simulink model "20240109_HVDCMMCInterconnection"  (R2023b)
settings: Solver=FixedStepDiscrete  StartTime=0.0  StopTime=2  FixedStep=Ts_Power  RelTol=1e-4  EnableMultiTasking=on
PreLoadFcn:
  | HVDCMMCInterconnectionParam
StartFcn:
  | tic
StopFcn:
  | toc
values from neighbouring files (symbols this model uses):
  C_PM = 1.758e-3    (= 0.001758)    [HVDCMMCInterconnectionParam.m]
  Cg = 50e-9    (= 5e-08)    [HVDCMMCInterconnectionParam.m]
  D_R = 0.001    [HVDCMMCInterconnectionParam.m]
  D_Rs = 1e8    (= 100000000)    [HVDCMMCInterconnectionParam.m]
  D_Vf = 0    [HVDCMMCInterconnectionParam.m]
  Fnom = 50    [HVDCMMCInterconnectionParam.m]
  HRM = 2    [HVDCMMCInterconnectionParam.m]
  Ki_Ireg = 6    [HVDCMMCInterconnectionParam.m]
  Ki_Preg = 1.0    (= 1)    [HVDCMMCInterconnectionParam.m]
  Ki_Qreg = 1.0    (= 1)    [HVDCMMCInterconnectionParam.m]
  Ki_VDCreg = 100    [HVDCMMCInterconnectionParam.m]
  Kp_Ireg = 0.6    [HVDCMMCInterconnectionParam.m]
  Kp_Preg = 0.5/3    (= 0.166666666667)    [HVDCMMCInterconnectionParam.m]
  Kp_Qreg = 0.5/3    (= 0.166666666667)    [HVDCMMCInterconnectionParam.m]
  Kp_VDCreg = 4    [HVDCMMCInterconnectionParam.m]
  L_cable = 15e-3    (= 0.015)    [HVDCMMCInterconnectionParam.m]
  Larm = Larm_pu*(Zb_ac/(2*pi*Fnom))    [HVDCMMCInterconnectionParam.m]
  Lff = Larm_pu/2    (= 0.075)    [HVDCMMCInterconnectionParam.m]
  Limits_Ireg = [ 2.0  -2.0]    [HVDCMMCInterconnectionParam.m]
  Limits_Preg = [ 1.2, 0.8 ]    [HVDCMMCInterconnectionParam.m]
  Limits_Qreg = [ 0.25, -0.25 ]    [HVDCMMCInterconnectionParam.m]
  Limits_VDCreg = [ 2.0  -2.0]    [HVDCMMCInterconnectionParam.m]
  Lxfo = 0.12    [HVDCMMCInterconnectionParam.m]
  Nb_PM = 36    [HVDCMMCInterconnectionParam.m]
  Pnom = 1000e6    (= 1000000000)    [HVDCMMCInterconnectionParam.m]
  R_cable = 0.5    [HVDCMMCInterconnectionParam.m]
  R_startup = 400    [HVDCMMCInterconnectionParam.m]
  Rarm = Rarm_pu*Zb_ac    [HVDCMMCInterconnectionParam.m]
  Rff = Rarm_pu/2    (= 0.00075)    [HVDCMMCInterconnectionParam.m]
  Rg = 100    [HVDCMMCInterconnectionParam.m]
  Rxfo = 0.003    [HVDCMMCInterconnectionParam.m]
  Slope_Pref = 0.5    [HVDCMMCInterconnectionParam.m]
  Slope_Qref = 0.5    [HVDCMMCInterconnectionParam.m]
  Slope_Vdc_ref = Vnom_dc/5    (= 128000)    [HVDCMMCInterconnectionParam.m]
  Tbrk1_On = 0.1    [HVDCMMCInterconnectionParam.m]
  Tbrk2_On = 1.0    (= 1)    [HVDCMMCInterconnectionParam.m]
  Tdeblock = 1.5    [HVDCMMCInterconnectionParam.m]
  Tfault = 9999    [HVDCMMCInterconnectionParam.m]
  Ton_Converter2 = 4    [HVDCMMCInterconnectionParam.m]
  Ton_PQreg = 4    [HVDCMMCInterconnectionParam.m]
  Ton_VDCreg = 1.5    [HVDCMMCInterconnectionParam.m]
  Ts = Ts_Control    (= 4e-05)    [HVDCMMCInterconnectionParam.m]
  Ts_Control = 40e-6    (= 4e-05)    [HVDCMMCInterconnectionParam.m]
  Ts_Power = 20e-6    (= 2e-05)    [HVDCMMCInterconnectionParam.m]
  Vb_ac = sqrt(2/3)*Vnom_sec    [HVDCMMCInterconnectionParam.m]
  Vb_dc = Vnom_dc    (= 640000)    [HVDCMMCInterconnectionParam.m]
  Vc0_PM = 0    [HVDCMMCInterconnectionParam.m]
  Vnom_dc = 640e3    (= 640000)    [HVDCMMCInterconnectionParam.m]
  Vnom_prim = 400e3    (= 400000)    [HVDCMMCInterconnectionParam.m]
  Vnom_sec = 333e3    (= 333000)    [HVDCMMCInterconnectionParam.m]
  w = 2*pi*Fnom    (= 314.159265359)    [HVDCMMCInterconnectionParam.m]
undefined symbols (not defined in the file or in its folder): DiscIntNeverNeededParam, gcbh, Pcc, S, sps_AC, sps_ACDC2, sps_rtmsupport
libraries: simulink x48, spsControlledVoltageSourceLib x30, spsCurrentMeasurementLib x30, MMC_Lib x30, spsDiodeLib x20, spsSeriesRLCBranchLib x14, powerlib_extras x12, spsVoltageMeasurementLib x12, spsSecondOrderFilterLib x8, spsabctodq0Lib x8, spsGroundLib x7, spsMeanLib x4
(part 6 of 9)

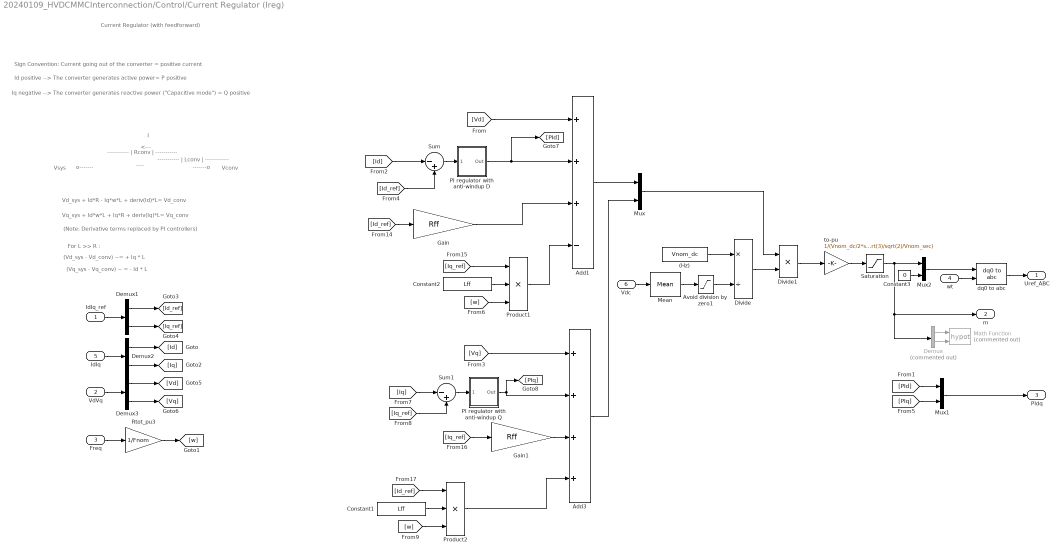
== system 20240109_HVDCMMCInterconnection/Control/Current Regulator (Ireg) ==
  note: -----------
      | | Lconv |
      | ------------
  note: <---
  note: -------o
  note: Vconv
  note: ----
  note: -----------
      | | Rconv |
      | -----------
  note: For L >> R :
  note: (Vq_sys - Vq_conv) ~ = - Id * L
  note: (Vd_sys - Vd_conv) ~= + Iq * L
  note: Id positive --> The converter generates active power= P positive
  note: Iq negative --> The converter generates reactive power ("Capacitive mode") = Q positive
  note: Sign Convention: Current going out of the converter = positive current
  note: Current Regulator
      | (with feedforward)
  note: Vq_sys + Id*w*L + Iq*R + deriv(Iq)*L= Vq_conv
  note: Vd_sys + Id*R - Iq*w*L + deriv(Id)*L= Vd_conv
  note: (Note: Derivative terms replaced by PI controllers)
  note: Vsys
  note: o-------
  note: I
  IdIq_ref : Inport  PortDimensions=2
  VdVq : Inport  Port=2  PortDimensions=2
  Freq : Inport  Port=3  PortDimensions=1
  wt : Inport  Port=4  PortDimensions=1
  IdIq : Inport  Port=5  PortDimensions=2
  Vdc : Inport  Port=6  PortDimensions=1
  " (Hz)" : Constant  Value=Vnom_dc  SampleTime=Ts
  Add1 : Sum  Inputs=+++-
  Add3 : Sum  Inputs=++++
  Avoid division by zero1 : Saturate  UpperLimit=Vnom_dc*1.25  LowerLimit=Vnom_dc*0.75
  Constant1 : Constant  Value=Lff  SampleTime=Ts_Control
  Constant2 : Constant  Value=Lff  SampleTime=Ts_Control
  Constant3 : Constant  Value=0  SampleTime=Ts
  Demux : Demux  Commented=on  Outputs=2
  Demux1 : Demux  Outputs=2
  Demux2 : Demux  Outputs=2
  Demux3 : Demux  Outputs=2
  Divide : Product  Inputs=*/
  Divide1 : Product  Inputs=**
  Gain : Gain  Gain=Rff
  Gain1 : Gain  Gain=Rff
  Math Function : Math  Commented=on  Operator=hypot  SignedPower=on
  Mean : spsMeanLib/Mean  Freq=Fnom/3  Vinit=Vnom_dc  Ts=Ts
  Mux : Mux  Inputs=2
  Mux1 : Mux  Inputs=2
  Mux2 : Mux  Inputs=[2 1]
  PI regulator with anti-windup D : Subsystem  DialogController=POWERSYS.PowerSysDialog  mask(Discrete PI Controller){Kp=Kp_Ireg, Ki=Ki_Ireg, Par_Limits=Limits_Ireg, Init=0, Ts=Ts}
      mask prompts: Kp "Proportional gain (Kp):"; Ki "Integral gain (Ki):"; Par_Limits "Output limits: [ Upper   Lower ]"; Init "Output initial value:"; Ts "Sample time:"
      mask help: This block implements a discrete PI controller.
      mask init:
      | UpperLimit=Par_Limits(1);
      | LowerLimit=Par_Limits(2);
      | power_initmask();
      mask Help: This block is part of a subset of blocks in the Extras library that does not have documentation associated with it, other than the block mask description.
      mask Display: disp('PI');
  PI regulator with anti-windup Q : Subsystem  DialogController=POWERSYS.PowerSysDialog  mask(Discrete PI Controller){Kp=Kp_Ireg, Ki=Ki_Ireg, Par_Limits=Limits_Ireg, Init=0, Ts=Ts}
      mask prompts: Kp "Proportional gain (Kp):"; Ki "Integral gain (Ki):"; Par_Limits "Output limits: [ Upper   Lower ]"; Init "Output initial value:"; Ts "Sample time:"
      mask help: This block implements a discrete PI controller.
      mask init:
      | UpperLimit=Par_Limits(1);
      | LowerLimit=Par_Limits(2);
      | power_initmask();
      mask Help: This block is part of a subset of blocks in the Extras library that does not have documentation associated with it, other than the block mask description.
      mask Display: disp('PI');
  Product1 : Product  Inputs=3  RndMeth=Zero
  Product2 : Product  Inputs=3  RndMeth=Zero
  Rtot_pu3 : Gain  Gain=1/Fnom  SaturateOnIntegerOverflow=on  OutDataTypeStr=Inherit: Same as input  ParamDataTypeStr=Inherit: Same as input
  Saturation : Saturate  UpperLimit=Limits_Ireg(1)  LowerLimit=Limits_Ireg(2)
  Sum : Sum  Inputs=|-+
  Sum1 : Sum  Inputs=|-+
  dq0 to abc : spsdq0toabcLib/dq0 to abc  Alignment=90 degrees behind phase A axis
  to-pu : Gain  Gain=1/(Vnom_dc/2*sqrt(3)/sqrt(2)/Vnom_sec)
  Uref_ABC : Outport
  m : Outport  Port=2
  PIdq : Outport  Port=3
  wires:
  wt/1 -> dq0 to abc/2
  to-pu/1 -> Saturation/1
  Mux/1 -> Divide1/1
  dq0 to abc/1 -> Uref_ABC/1
  Divide/1 -> Divide1/2
  Mean/1 -> Avoid division by zero1/1
  Divide1/1 -> to-pu/1
  " (Hz)"/1 -> Divide/1
  Vdc/1 -> Mean/1
  Avoid division by zero1/1 -> Divide/2
  Mux1/1 -> PIdq/1
  Constant3/1 -> Mux2/2
  Mux2/1 -> dq0 to abc/1
  Demux/2 -> Math Function/2
  Demux/1 -> Math Function/1
  Saturation/1 -> Mux2/1, m/1, Demux/1
  PI regulator with anti-windup D/1(Out) -> [PId], Add1/2
  PI regulator with anti-windup Q/1(Out) -> [PIq], Add3/2
  [Vd] -> Add1/1
  Product1/1 -> Add1/4
  Gain/1 -> Add1/3
  Gain1/1 -> Add3/3
  Product2/1 -> Add3/4
  [Vq] -> Add3/1
  Demux2/1 -> [Id]
  IdIq/1 -> Demux2/1
  [Id_ref] -> Product2/1
  [Iq_ref] -> Gain1/1
  [Iq_ref] -> Product1/1
  [Id_ref] -> Gain/1
  [Id] -> Sum/1
  [Iq] -> Sum1/1
  Demux2/2 -> [Iq]
  [PIq] -> Mux1/2
  [PId] -> Mux1/1
  [w] -> Product1/3
  Constant2/1 -> Product1/2
  [w] -> Product2/3
  Constant1/1 -> Product2/2
  [Iq_ref] -> Sum1/2
  Sum1/1 -> PI regulator with anti-windup Q/1(Error)
  [Id_ref] -> Sum/2
  Sum/1 -> PI regulator with anti-windup D/1(Error)
  VdVq/1 -> Demux3/1
  Demux3/2 -> [Vq]
  Demux3/1 -> [Vd]
  IdIq_ref/1 -> Demux1/1
  Demux1/2 -> [Iq_ref]
  Demux1/1 -> [Id_ref]
  Rtot_pu3/1 -> [w]
  Freq/1 -> Rtot_pu3/1
  Add1/1 -> Mux/1
  Add3/1 -> Mux/2

== system 20240109_HVDCMMCInterconnection/Control/DC Voltage Regulator (VDCreg) ==
  note: VDC Regulator
  Vdc_ref : Inport  PortDimensions=1
  On : Inport  Port=2  PortDimensions=1
  Vdc_meas : Inport  Port=3  PortDimensions=1
  Discrete-Time Integrator : DiscreteIntegrator  SampleTime=Ts  LimitOutput=on  UpperSaturationLimit=Limits_VDCreg(1)  LowerSaturationLimit=Limits_VDCreg(2)  ICPrevOutput=DiscIntNeverNeededParam  ICPrevScaledInput=DiscIntNeverNeededParam
  Product : Product  RndMeth=Zero
  Product1 : Product  RndMeth=Zero
  Rtot_pu2 : Gain  Gain=1/Vnom_dc  SaturateOnIntegerOverflow=on  OutDataTypeStr=Inherit: Same as input  ParamDataTypeStr=Inherit: Same as input
  Saturation2 : Saturate  UpperLimit=Limits_VDCreg(1)  LowerLimit=Limits_VDCreg(2)  SampleTime=Ts
  Sum : Sum  Inputs=|+-
  Sum6 : Sum  InputSameDT=on  SaturateOnIntegerOverflow=on  SampleTime=Ts  OutDataTypeStr=Inherit: Same as first input
  Switch1 : Switch  Criteria=u2 ~= 0  Threshold=0.5  OutDataTypeStr=double  SaturateOnIntegerOverflow=off  InputSameDT=off
  VdcNom_SM : Constant  Value=Kp_VDCreg
  VdcNom_SM1 : Constant  Value=Ki_VDCreg
  Zero-Order Hold : ZeroOrderHold  SampleTime=Ts
  Id_ref : Outport
  wires:
  Rtot_pu2/1 -> Product/2, Product1/2
  Saturation2/1 -> Id_ref/1
  VdcNom_SM/1 -> Product1/1
  Product/1 -> Discrete-Time Integrator/1
  Product1/1 -> Zero-Order Hold/1
  VdcNom_SM1/1 -> Product/1
  Sum6/1 -> Saturation2/1
  Discrete-Time Integrator/1 -> Sum6/2
  Zero-Order Hold/1 -> Sum6/1
  Vdc_ref/1 -> Sum/2, Switch1/3
  Switch1/1 -> Sum/1
  On/1 -> Switch1/2
  Sum/1 -> Rtot_pu2/1
  Vdc_meas/1 -> Switch1/1

== system 20240109_HVDCMMCInterconnection/Control/PLL, Measurements and Transformation ==
  note: P (pu) = Vd*Id + Vq*Iq
  note: Q (pu) = Vq*Id - Vd*Iq
  note: P positive = Converter generates active power (Inverter Mode)
  note: Q positive = Converter generates reactive power (Capacitive Mode)
  Vabc : Inport  PortDimensions=3
  Iabc : Inport  Port=2  PortDimensions=3
  Add : Sum  Inputs=1
  Demux : Demux  Outputs=2
  Discrete Mean value : powerlib_extras/Discrete Measurements/Discrete  Mean value  Freq=Fnom  Vinit=0  Ts=Ts
  Discrete Mean value1 : powerlib_extras/Discrete Measurements/Discrete  Mean value  Freq=Fnom  Vinit=0  Ts=Ts
  I->pu2 : Gain  Gain=sqrt(3)*Vnom_sec/sqrt(2)/Pnom  SaturateOnIntegerOverflow=on  OutDataTypeStr=Inherit: Same as input  ParamDataTypeStr=Inherit: Same as input
  PLL (3ph) : spsPLL3phLib/PLL (3ph)  Fmin=0.9*Fnom  Par_Init=[0, Fnom]  ParK=[180, 3200, 1]  TcD=1e-4  MaxRateChangeFreq=12  FilterCutOffFreq=25  Ts=Ts  AGC=on
  Product : Product  RndMeth=Zero
  Product1 : Product  RndMeth=Zero
  Second-Order Filter : spsSecondOrderFilterLib/Second-Order Filter  FilterType=Lowpass  Fo=Fn_filter  Zeta=Zeta_filter  Ts=Ts  Initialize=off  Vac_Init="[0,  0,  60]"  Vdc_Init=0  PlotResponse=off  FreqRange=[0, 500, 1]
  Second-Order Filter1 : spsSecondOrderFilterLib/Second-Order Filter  FilterType=Lowpass  Fo=Fn_filter  Zeta=Zeta_filter  Ts=Ts  Initialize=off  Vac_Init="[0,  0,  60]"  Vdc_Init=0  PlotResponse=off  FreqRange=[0, 500, 1]
  Selector3 : Selector  InputPortWidth=2  IndexOptions=Index vector (dialog)  Indices=[2 1]  OutputSizes=1
  Selector4 : Selector  InputPortWidth=3  IndexOptions=Index vector (dialog)  Indices=[1 2]  OutputSizes=1
  Selector5 : Selector  InputPortWidth=3  IndexOptions=Index vector (dialog)  Indices=[1 2]  OutputSizes=1
  Subtract : Sum  Inputs=+-
  V->pu1 : Gain  Gain=1/(Vnom_sec/sqrt(3)*sqrt(2))  SaturateOnIntegerOverflow=on  OutDataTypeStr=Inherit: Same as input  ParamDataTypeStr=Inherit: Same as input
  abc to dq0 : spsabctodq0Lib/abc to dq0  Alignment=90 degrees behind phase A axis
  abc to dq1 : spsabctodq0Lib/abc to dq0  Alignment=90 degrees behind phase A axis
  Freq : Outport
  wt : Outport  Port=2
  IdIq : Outport  Port=3
  P : Outport  Port=4
  Q : Outport  Port=5
  VdVq : Outport  Port=6
  wires:
  Selector3/1 -> Product1/1
  Discrete Mean value1/1 -> Q/1
  Discrete Mean value/1 -> P/1
  Second-Order Filter/1 -> VdVq/1, Product/1, Selector3/1
  Second-Order Filter1/1 -> IdIq/1, Product1/2, Product/2
  Product/1 -> Add/1
  Product1/1 -> Demux/1
  Demux/1 -> Subtract/1
  Demux/2 -> Subtract/2
  Add/1 -> Discrete Mean value/1
  Subtract/1 -> Discrete Mean value1/1
  abc to dq0/1 -> Selector4/1
  PLL (3ph)/1 -> Freq/1
  V->pu1/1 -> abc to dq0/1, PLL (3ph)/1
  Vabc/1 -> V->pu1/1
  PLL (3ph)/2 -> wt/1, abc to dq1/2, abc to dq0/2
  Iabc/1 -> I->pu2/1
  abc to dq1/1 -> Selector5/1
  I->pu2/1 -> abc to dq1/1
  Selector4/1 -> Second-Order Filter/1
  Selector5/1 -> Second-Order Filter1/1

== system 20240109_HVDCMMCInterconnection/Control/Reactive Power Regulator ==
  note: Reactive Power Regulator
  note: If PLL sync on Vprim --> Vq=0 --> Id = P/Vd et Iq = -1.0 * Q/Vd
  note: Q (pu) = Vq*Id - Vd*Iq (valid only for balanced & harmonics-free values)
  note: P (pu) = Vd*Id + Vq*Iq (Zero-sequence is not taken into account)
  On : Inport  PortDimensions=1
  Qref : Inport  Port=2  PortDimensions=1
  Qmes : Inport  Port=3  PortDimensions=1
  VdVq_mes : Inport  Port=4  PortDimensions=2
  Add2 : Sum
  Discrete Mean value1 : powerlib_extras/Discrete Measurements/Discrete  Mean value  Freq=Fnom  Vinit=0  Ts=Ts
  Discrete-Time Integrator : DiscreteIntegrator  SampleTime=Ts  LimitOutput=on  UpperSaturationLimit=Limits_Qreg(1)  LowerSaturationLimit=Limits_Qreg(2)  ICPrevOutput=DiscIntNeverNeededParam  ICPrevScaledInput=DiscIntNeverNeededParam
  Divide : Product  Inputs=*/
  Product : Product  RndMeth=Zero
  Product1 : Product  RndMeth=Zero
  Rtot_pu1 : Gain  Gain=-1  SaturateOnIntegerOverflow=on  OutDataTypeStr=Inherit: Same as input  ParamDataTypeStr=Inherit: Same as input
  Rtot_pu2 : Gain  Gain=-1  SaturateOnIntegerOverflow=on  OutDataTypeStr=Inherit: Same as input  ParamDataTypeStr=Inherit: Same as input
  Saturation : Saturate  UpperLimit=Limits_Qreg(1)  LowerLimit=Limits_Qreg(2)
  Saturation1 : Saturate  UpperLimit=2  LowerLimit=1e-6
  Saturation2 : Saturate  UpperLimit=Limits_Qreg(1)  LowerLimit=Limits_Qreg(2)
  Selector : Selector  InputPortWidth=2  IndexOptions=Index vector (dialog)  Indices=[1]  OutputSizes=1
  Sum : Sum  Inputs=|-+
  Sum6 : Sum  InputSameDT=on  SaturateOnIntegerOverflow=on  SampleTime=Ts  OutDataTypeStr=Inherit: Same as first input
  Switch1 : Switch  Criteria=u2 ~= 0  Threshold=0.5  OutDataTypeStr=double  SaturateOnIntegerOverflow=off  InputSameDT=off
  VdcNom_SM : Constant  Value=Kp_Qreg
  VdcNom_SM1 : Constant  Value=Ki_Qreg
  Zero-Order Hold : ZeroOrderHold  SampleTime=Ts
  Iq_ref : Outport
  wires:
  Saturation2/1 -> Rtot_pu1/1
  Saturation/1 -> Iq_ref/1
  Rtot_pu2/1 -> Add2/2
  Rtot_pu1/1 -> Add2/1
  Sum6/1 -> Saturation2/1
  Switch1/1 -> Product1/2, Product/2
  Sum/1 -> Switch1/1
  On/1 -> Switch1/2
  Add2/1 -> Saturation/1
  Product/1 -> Discrete-Time Integrator/1
  Product1/1 -> Zero-Order Hold/1
  VdcNom_SM/1 -> Product1/1
  VdcNom_SM1/1 -> Product/1
  Discrete-Time Integrator/1 -> Sum6/2
  Zero-Order Hold/1 -> Sum6/1
  Discrete Mean value1/1 -> Saturation1/1
  Saturation1/1 -> Divide/2
  Divide/1 -> Rtot_pu2/1
  Selector/1 -> Discrete Mean value1/1
  VdVq_mes/1 -> Selector/1
  Qmes/1 -> Sum/1
  Qref/1 -> Divide/1, Switch1/3, Sum/2

== system 20240109_HVDCMMCInterconnection/Control1/Active Power Regulator (Preg) ==
  note: Active Power Regulator
  Pmeas : Inport  PortDimensions=1
  Pref : Inport  Port=2  PortDimensions=1  SampleTime=Ts
  On : Inport  Port=3  PortDimensions=1  SampleTime=Ts
  Discrete-Time Integrator : DiscreteIntegrator  InitialCondition=1  SampleTime=Ts  LimitOutput=on  UpperSaturationLimit=Limits_Preg(1)  LowerSaturationLimit=Limits_Preg(2)  ICPrevOutput=DiscIntNeverNeededParam  ICPrevScaledInput=DiscIntNeverNeededParam
  Product : Product  RndMeth=Zero
  Product1 : Product  RndMeth=Zero
  Product2 : Product
  Saturation2 : Saturate  UpperLimit=Limits_Preg(1)  LowerLimit=Limits_Preg(2)  SampleTime=Ts
  Sum : Sum  Inputs=|+-
  Sum6 : Sum  InputSameDT=on  SaturateOnIntegerOverflow=on  SampleTime=Ts  OutDataTypeStr=Inherit: Same as first input
  Switch1 : Switch  Criteria=u2 ~= 0  Threshold=0.5  OutDataTypeStr=double  SaturateOnIntegerOverflow=off  InputSameDT=off
  VdcNom_SM : Constant  Value=Kp_Preg  SampleTime=Ts
  VdcNom_SM1 : Constant  Value=Ki_Preg  SampleTime=Ts
  VdcNom_SM2 : Constant  Value=Vnom_dc  SampleTime=Ts
  Zero-Order Hold : ZeroOrderHold  SampleTime=Ts
  Vdc_ref : Outport  SampleTime=Ts
  wires:
  Product2/1 -> Vdc_ref/1
  VdcNom_SM2/1 -> Product2/2
  Pmeas/1 -> Switch1/1
  On/1 -> Switch1/2
  Switch1/1 -> Sum/1
  Pref/1 -> Switch1/3, Sum/2
  Zero-Order Hold/1 -> Sum6/1
  Discrete-Time Integrator/1 -> Sum6/2
  Sum6/1 -> Saturation2/1
  VdcNom_SM1/1 -> Product/1
  Product1/1 -> Zero-Order Hold/1
  Product/1 -> Discrete-Time Integrator/1
  VdcNom_SM/1 -> Product1/1
  Saturation2/1 -> Product2/1
  Sum/1 -> Product1/2, Product/2

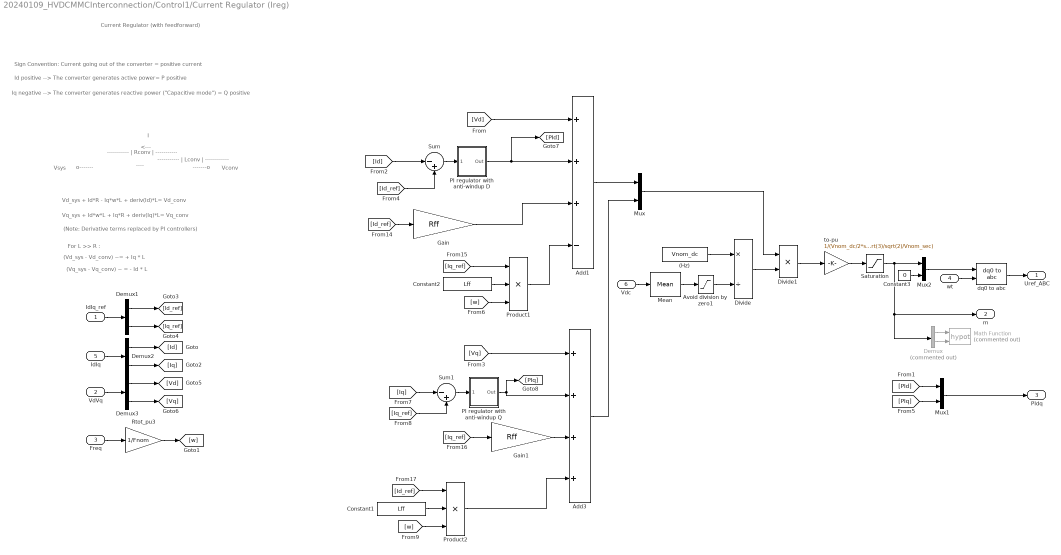
== system 20240109_HVDCMMCInterconnection/Control1/Current Regulator (Ireg) ==
  note: -----------
      | | Lconv |
      | ------------
  note: <---
  note: -------o
  note: Vconv
  note: ----
  note: -----------
      | | Rconv |
      | -----------
  note: For L >> R :
  note: (Vq_sys - Vq_conv) ~ = - Id * L
  note: (Vd_sys - Vd_conv) ~= + Iq * L
  note: Id positive --> The converter generates active power= P positive
  note: Iq negative --> The converter generates reactive power ("Capacitive mode") = Q positive
  note: Sign Convention: Current going out of the converter = positive current
  note: Current Regulator
      | (with feedforward)
  note: Vq_sys + Id*w*L + Iq*R + deriv(Iq)*L= Vq_conv
  note: Vd_sys + Id*R - Iq*w*L + deriv(Id)*L= Vd_conv
  note: (Note: Derivative terms replaced by PI controllers)
  note: Vsys
  note: o-------
  note: I
  IdIq_ref : Inport  PortDimensions=2
  VdVq : Inport  Port=2  PortDimensions=2
  Freq : Inport  Port=3  PortDimensions=1
  wt : Inport  Port=4  PortDimensions=1
  IdIq : Inport  Port=5  PortDimensions=2
  Vdc : Inport  Port=6  PortDimensions=1
  " (Hz)" : Constant  Value=Vnom_dc  SampleTime=Ts
  Add1 : Sum  Inputs=+++-
  Add3 : Sum  Inputs=++++
  Avoid division by zero1 : Saturate  UpperLimit=Vnom_dc*1.25  LowerLimit=Vnom_dc*0.75
  Constant1 : Constant  Value=Lff  SampleTime=Ts_Control
  Constant2 : Constant  Value=Lff  SampleTime=Ts_Control
  Constant3 : Constant  Value=0  SampleTime=Ts
  Demux : Demux  Commented=on  Outputs=2
  Demux1 : Demux  Outputs=2
  Demux2 : Demux  Outputs=2
  Demux3 : Demux  Outputs=2
  Divide : Product  Inputs=*/
  Divide1 : Product  Inputs=**
  Gain : Gain  Gain=Rff
  Gain1 : Gain  Gain=Rff
  Math Function : Math  Commented=on  Operator=hypot  SignedPower=on
  Mean : spsMeanLib/Mean  Freq=Fnom/3  Vinit=Vnom_dc  Ts=Ts
  Mux : Mux  Inputs=2
  Mux1 : Mux  Inputs=2
  Mux2 : Mux  Inputs=[2 1]
  PI regulator with anti-windup D : Subsystem  DialogController=POWERSYS.PowerSysDialog  mask(Discrete PI Controller){Kp=Kp_Ireg, Ki=Ki_Ireg, Par_Limits=Limits_Ireg, Init=0, Ts=Ts}
      mask prompts: Kp "Proportional gain (Kp):"; Ki "Integral gain (Ki):"; Par_Limits "Output limits: [ Upper   Lower ]"; Init "Output initial value:"; Ts "Sample time:"
      mask help: This block implements a discrete PI controller.
      mask init:
      | UpperLimit=Par_Limits(1);
      | LowerLimit=Par_Limits(2);
      | power_initmask();
      mask Help: This block is part of a subset of blocks in the Extras library that does not have documentation associated with it, other than the block mask description.
      mask Display: disp('PI');
  PI regulator with anti-windup Q : Subsystem  DialogController=POWERSYS.PowerSysDialog  mask(Discrete PI Controller){Kp=Kp_Ireg, Ki=Ki_Ireg, Par_Limits=Limits_Ireg, Init=0, Ts=Ts}
      mask prompts: Kp "Proportional gain (Kp):"; Ki "Integral gain (Ki):"; Par_Limits "Output limits: [ Upper   Lower ]"; Init "Output initial value:"; Ts "Sample time:"
      mask help: This block implements a discrete PI controller.
      mask init:
      | UpperLimit=Par_Limits(1);
      | LowerLimit=Par_Limits(2);
      | power_initmask();
      mask Help: This block is part of a subset of blocks in the Extras library that does not have documentation associated with it, other than the block mask description.
      mask Display: disp('PI');
  Product1 : Product  Inputs=3  RndMeth=Zero
  Product2 : Product  Inputs=3  RndMeth=Zero
  Rtot_pu3 : Gain  Gain=1/Fnom  SaturateOnIntegerOverflow=on  OutDataTypeStr=Inherit: Same as input  ParamDataTypeStr=Inherit: Same as input
  Saturation : Saturate  UpperLimit=Limits_Ireg(1)  LowerLimit=Limits_Ireg(2)
  Sum : Sum  Inputs=|-+
  Sum1 : Sum  Inputs=|-+
  dq0 to abc : spsdq0toabcLib/dq0 to abc  Alignment=90 degrees behind phase A axis
  to-pu : Gain  Gain=1/(Vnom_dc/2*sqrt(3)/sqrt(2)/Vnom_sec)
  Uref_ABC : Outport
  m : Outport  Port=2
  PIdq : Outport  Port=3
  wires:
  wt/1 -> dq0 to abc/2
  to-pu/1 -> Saturation/1
  Mux/1 -> Divide1/1
  dq0 to abc/1 -> Uref_ABC/1
  Divide/1 -> Divide1/2
  Mean/1 -> Avoid division by zero1/1
  Divide1/1 -> to-pu/1
  " (Hz)"/1 -> Divide/1
  Vdc/1 -> Mean/1
  Avoid division by zero1/1 -> Divide/2
  Mux1/1 -> PIdq/1
  Constant3/1 -> Mux2/2
  Mux2/1 -> dq0 to abc/1
  Demux/2 -> Math Function/2
  Demux/1 -> Math Function/1
  Saturation/1 -> Mux2/1, m/1, Demux/1
  PI regulator with anti-windup D/1(Out) -> [PId], Add1/2
  PI regulator with anti-windup Q/1(Out) -> [PIq], Add3/2
  [Vd] -> Add1/1
  Product1/1 -> Add1/4
  Gain/1 -> Add1/3
  Gain1/1 -> Add3/3
  Product2/1 -> Add3/4
  [Vq] -> Add3/1
  Demux2/1 -> [Id]
  IdIq/1 -> Demux2/1
  [Id_ref] -> Product2/1
  [Iq_ref] -> Gain1/1
  [Iq_ref] -> Product1/1
  [Id_ref] -> Gain/1
  [Id] -> Sum/1
  [Iq] -> Sum1/1
  Demux2/2 -> [Iq]
  [PIq] -> Mux1/2
  [PId] -> Mux1/1
  [w] -> Product1/3
  Constant2/1 -> Product1/2
  [w] -> Product2/3
  Constant1/1 -> Product2/2
  [Iq_ref] -> Sum1/2
  Sum1/1 -> PI regulator with anti-windup Q/1(Error)
  [Id_ref] -> Sum/2
  Sum/1 -> PI regulator with anti-windup D/1(Error)
  VdVq/1 -> Demux3/1
  Demux3/2 -> [Vq]
  Demux3/1 -> [Vd]
  IdIq_ref/1 -> Demux1/1
  Demux1/2 -> [Iq_ref]
  Demux1/1 -> [Id_ref]
  Rtot_pu3/1 -> [w]
  Freq/1 -> Rtot_pu3/1
  Add1/1 -> Mux/1
  Add3/1 -> Mux/2

== system 20240109_HVDCMMCInterconnection/Control1/DC Voltage Regulator (VDCreg) ==
  note: VDC Regulator
  Vdc_ref : Inport  PortDimensions=1
  On : Inport  Port=2  PortDimensions=1
  Vdc_meas : Inport  Port=3  PortDimensions=1
  Discrete-Time Integrator : DiscreteIntegrator  SampleTime=Ts  LimitOutput=on  UpperSaturationLimit=Limits_VDCreg(1)  LowerSaturationLimit=Limits_VDCreg(2)  ICPrevOutput=DiscIntNeverNeededParam  ICPrevScaledInput=DiscIntNeverNeededParam
  Product : Product  RndMeth=Zero
  Product1 : Product  RndMeth=Zero
  Rtot_pu2 : Gain  Gain=1/Vnom_dc  SaturateOnIntegerOverflow=on  OutDataTypeStr=Inherit: Same as input  ParamDataTypeStr=Inherit: Same as input
  Saturation2 : Saturate  UpperLimit=Limits_VDCreg(1)  LowerLimit=Limits_VDCreg(2)  SampleTime=Ts
  Sum : Sum  Inputs=|+-
  Sum6 : Sum  InputSameDT=on  SaturateOnIntegerOverflow=on  SampleTime=Ts  OutDataTypeStr=Inherit: Same as first input
  Switch1 : Switch  Criteria=u2 ~= 0  Threshold=0.5  OutDataTypeStr=double  SaturateOnIntegerOverflow=off  InputSameDT=off
  VdcNom_SM : Constant  Value=Kp_VDCreg
  VdcNom_SM1 : Constant  Value=Ki_VDCreg
  Zero-Order Hold : ZeroOrderHold  SampleTime=Ts
  Id_ref : Outport
  wires:
  Rtot_pu2/1 -> Product/2, Product1/2
  Saturation2/1 -> Id_ref/1
  VdcNom_SM/1 -> Product1/1
  Product/1 -> Discrete-Time Integrator/1
  Product1/1 -> Zero-Order Hold/1
  VdcNom_SM1/1 -> Product/1
  Sum6/1 -> Saturation2/1
  Discrete-Time Integrator/1 -> Sum6/2
  Zero-Order Hold/1 -> Sum6/1
  Vdc_ref/1 -> Sum/2, Switch1/3
  Switch1/1 -> Sum/1
  On/1 -> Switch1/2
  Sum/1 -> Rtot_pu2/1
  Vdc_meas/1 -> Switch1/1

== system 20240109_HVDCMMCInterconnection/Control1/PLL, Measurements and Transformation ==
  note: P (pu) = Vd*Id + Vq*Iq
  note: Q (pu) = Vq*Id - Vd*Iq
  note: P positive = Converter generates active power (Inverter Mode)
  note: Q positive = Converter generates reactive power (Capacitive Mode)
  Vabc : Inport  PortDimensions=3
  Iabc : Inport  Port=2  PortDimensions=3
  Add : Sum  Inputs=1
  Demux : Demux  Outputs=2
  Discrete Mean value : powerlib_extras/Discrete Measurements/Discrete  Mean value  Freq=Fnom  Vinit=0  Ts=Ts
  Discrete Mean value1 : powerlib_extras/Discrete Measurements/Discrete  Mean value  Freq=Fnom  Vinit=0  Ts=Ts
  I->pu2 : Gain  Gain=sqrt(3)*Vnom_sec/sqrt(2)/Pnom  SaturateOnIntegerOverflow=on  OutDataTypeStr=Inherit: Same as input  ParamDataTypeStr=Inherit: Same as input
  PLL (3ph) : spsPLL3phLib/PLL (3ph)  Fmin=0.9*Fnom  Par_Init=[0, Fnom]  ParK=[180, 3200, 1]  TcD=1e-4  MaxRateChangeFreq=12  FilterCutOffFreq=25  Ts=Ts  AGC=on
  Product : Product  RndMeth=Zero
  Product1 : Product  RndMeth=Zero
  Second-Order Filter : spsSecondOrderFilterLib/Second-Order Filter  FilterType=Lowpass  Fo=Fn_filter  Zeta=Zeta_filter  Ts=Ts  Initialize=off  Vac_Init="[0,  0,  60]"  Vdc_Init=0  PlotResponse=off  FreqRange=[0, 500, 1]
  Second-Order Filter1 : spsSecondOrderFilterLib/Second-Order Filter  FilterType=Lowpass  Fo=Fn_filter  Zeta=Zeta_filter  Ts=Ts  Initialize=off  Vac_Init="[0,  0,  60]"  Vdc_Init=0  PlotResponse=off  FreqRange=[0, 500, 1]
  Selector3 : Selector  InputPortWidth=2  IndexOptions=Index vector (dialog)  Indices=[2 1]  OutputSizes=1
  Selector4 : Selector  InputPortWidth=3  IndexOptions=Index vector (dialog)  Indices=[1 2]  OutputSizes=1
  Selector5 : Selector  InputPortWidth=3  IndexOptions=Index vector (dialog)  Indices=[1 2]  OutputSizes=1
  Subtract : Sum  Inputs=+-
  V->pu1 : Gain  Gain=1/(Vnom_sec/sqrt(3)*sqrt(2))  SaturateOnIntegerOverflow=on  OutDataTypeStr=Inherit: Same as input  ParamDataTypeStr=Inherit: Same as input
  abc to dq0 : spsabctodq0Lib/abc to dq0  Alignment=90 degrees behind phase A axis
  abc to dq1 : spsabctodq0Lib/abc to dq0  Alignment=90 degrees behind phase A axis
  Freq : Outport
  wt : Outport  Port=2
  IdIq : Outport  Port=3
  P : Outport  Port=4
  Q : Outport  Port=5
  VdVq : Outport  Port=6
  wires:
  Selector3/1 -> Product1/1
  Discrete Mean value1/1 -> Q/1
  Discrete Mean value/1 -> P/1
  Second-Order Filter/1 -> VdVq/1, Product/1, Selector3/1
  Second-Order Filter1/1 -> IdIq/1, Product1/2, Product/2
  Product/1 -> Add/1
  Product1/1 -> Demux/1
  Demux/1 -> Subtract/1
  Demux/2 -> Subtract/2
  Add/1 -> Discrete Mean value/1
  Subtract/1 -> Discrete Mean value1/1
  abc to dq0/1 -> Selector4/1
  PLL (3ph)/1 -> Freq/1
  V->pu1/1 -> abc to dq0/1, PLL (3ph)/1
  Vabc/1 -> V->pu1/1
  PLL (3ph)/2 -> wt/1, abc to dq1/2, abc to dq0/2
  Iabc/1 -> I->pu2/1
  abc to dq1/1 -> Selector5/1
  I->pu2/1 -> abc to dq1/1
  Selector4/1 -> Second-Order Filter/1
  Selector5/1 -> Second-Order Filter1/1

== system 20240109_HVDCMMCInterconnection/Control1/Reactive Power Regulator ==
  note: Reactive Power Regulator
  note: If PLL sync on Vprim --> Vq=0 --> Id = P/Vd et Iq = -1.0 * Q/Vd
  note: Q (pu) = Vq*Id - Vd*Iq (valid only for balanced & harmonics-free values)
  note: P (pu) = Vd*Id + Vq*Iq (Zero-sequence is not taken into account)
  On : Inport  PortDimensions=1
  Qref : Inport  Port=2  PortDimensions=1
  Qmes : Inport  Port=3  PortDimensions=1
  VdVq_mes : Inport  Port=4  PortDimensions=2
  Add2 : Sum
  Discrete Mean value1 : powerlib_extras/Discrete Measurements/Discrete  Mean value  Freq=Fnom  Vinit=0  Ts=Ts
  Discrete-Time Integrator : DiscreteIntegrator  SampleTime=Ts  LimitOutput=on  UpperSaturationLimit=Limits_Qreg(1)  LowerSaturationLimit=Limits_Qreg(2)  ICPrevOutput=DiscIntNeverNeededParam  ICPrevScaledInput=DiscIntNeverNeededParam
  Divide : Product  Inputs=*/
  Product : Product  RndMeth=Zero
  Product1 : Product  RndMeth=Zero
  Rtot_pu1 : Gain  Gain=-1  SaturateOnIntegerOverflow=on  OutDataTypeStr=Inherit: Same as input  ParamDataTypeStr=Inherit: Same as input
  Rtot_pu2 : Gain  Gain=-1  SaturateOnIntegerOverflow=on  OutDataTypeStr=Inherit: Same as input  ParamDataTypeStr=Inherit: Same as input
  Saturation : Saturate  UpperLimit=Limits_Qreg(1)  LowerLimit=Limits_Qreg(2)
  Saturation1 : Saturate  UpperLimit=2  LowerLimit=1e-6
  Saturation2 : Saturate  UpperLimit=Limits_Qreg(1)  LowerLimit=Limits_Qreg(2)
  Selector : Selector  InputPortWidth=2  IndexOptions=Index vector (dialog)  Indices=[1]  OutputSizes=1
  Sum : Sum  Inputs=|-+
  Sum6 : Sum  InputSameDT=on  SaturateOnIntegerOverflow=on  SampleTime=Ts  OutDataTypeStr=Inherit: Same as first input
  Switch1 : Switch  Criteria=u2 ~= 0  Threshold=0.5  OutDataTypeStr=double  SaturateOnIntegerOverflow=off  InputSameDT=off
  VdcNom_SM : Constant  Value=Kp_Qreg
  VdcNom_SM1 : Constant  Value=Ki_Qreg
  Zero-Order Hold : ZeroOrderHold  SampleTime=Ts
  Iq_ref : Outport
  wires:
  Saturation2/1 -> Rtot_pu1/1
  Saturation/1 -> Iq_ref/1
  Rtot_pu2/1 -> Add2/2
  Rtot_pu1/1 -> Add2/1
  Sum6/1 -> Saturation2/1
  Switch1/1 -> Product1/2, Product/2
  Sum/1 -> Switch1/1
  On/1 -> Switch1/2
  Add2/1 -> Saturation/1
  Product/1 -> Discrete-Time Integrator/1
  Product1/1 -> Zero-Order Hold/1
  VdcNom_SM/1 -> Product1/1
  VdcNom_SM1/1 -> Product/1
  Discrete-Time Integrator/1 -> Sum6/2
  Zero-Order Hold/1 -> Sum6/1
  Discrete Mean value1/1 -> Saturation1/1
  Saturation1/1 -> Divide/2
  Divide/1 -> Rtot_pu2/1
  Selector/1 -> Discrete Mean value1/1
  VdVq_mes/1 -> Selector/1
  Qmes/1 -> Sum/1
  Qref/1 -> Divide/1, Switch1/3, Sum/2

== system 20240109_HVDCMMCInterconnection/Control2/Active Power Regulator (Preg) ==
  note: Active Power Regulator
  Pmeas : Inport  PortDimensions=1
  Pref : Inport  Port=2  PortDimensions=1  SampleTime=Ts
  On : Inport  Port=3  PortDimensions=1  SampleTime=Ts
  Discrete-Time Integrator : DiscreteIntegrator  InitialCondition=1  SampleTime=Ts  LimitOutput=on  UpperSaturationLimit=Limits_Preg(1)  LowerSaturationLimit=Limits_Preg(2)  ICPrevOutput=DiscIntNeverNeededParam  ICPrevScaledInput=DiscIntNeverNeededParam
  Product : Product  RndMeth=Zero
  Product1 : Product  RndMeth=Zero
  Product2 : Product
  Saturation2 : Saturate  UpperLimit=Limits_Preg(1)  LowerLimit=Limits_Preg(2)  SampleTime=Ts
  Sum : Sum  Inputs=|+-
  Sum6 : Sum  InputSameDT=on  SaturateOnIntegerOverflow=on  SampleTime=Ts  OutDataTypeStr=Inherit: Same as first input
  Switch1 : Switch  Criteria=u2 ~= 0  Threshold=0.5  OutDataTypeStr=double  SaturateOnIntegerOverflow=off  InputSameDT=off
  VdcNom_SM : Constant  Value=Kp_Preg  SampleTime=Ts
  VdcNom_SM1 : Constant  Value=Ki_Preg  SampleTime=Ts
  VdcNom_SM2 : Constant  Value=Vnom_dc  SampleTime=Ts
  Zero-Order Hold : ZeroOrderHold  SampleTime=Ts
  Vdc_ref : Outport  SampleTime=Ts
  wires:
  Product2/1 -> Vdc_ref/1
  VdcNom_SM2/1 -> Product2/2
  Pmeas/1 -> Switch1/1
  On/1 -> Switch1/2
  Switch1/1 -> Sum/1
  Pref/1 -> Switch1/3, Sum/2
  Zero-Order Hold/1 -> Sum6/1
  Discrete-Time Integrator/1 -> Sum6/2
  Sum6/1 -> Saturation2/1
  VdcNom_SM1/1 -> Product/1
  Product1/1 -> Zero-Order Hold/1
  Product/1 -> Discrete-Time Integrator/1
  VdcNom_SM/1 -> Product1/1
  Saturation2/1 -> Product2/1
  Sum/1 -> Product1/2, Product/2

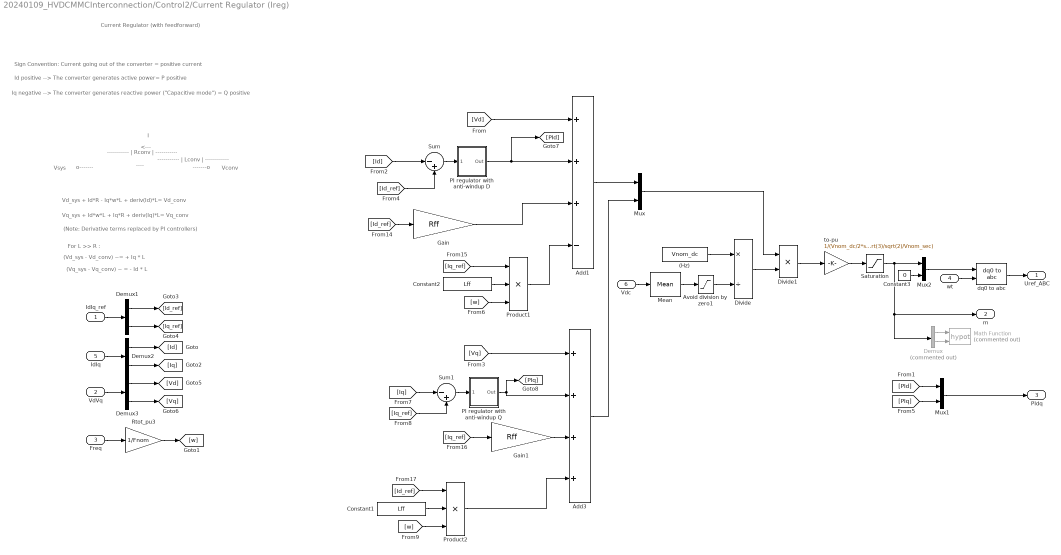
== system 20240109_HVDCMMCInterconnection/Control2/Current Regulator (Ireg) ==
  note: -----------
      | | Lconv |
      | ------------
  note: <---
  note: -------o
  note: Vconv
  note: ----
  note: -----------
      | | Rconv |
      | -----------
  note: For L >> R :
  note: (Vq_sys - Vq_conv) ~ = - Id * L
  note: (Vd_sys - Vd_conv) ~= + Iq * L
  note: Id positive --> The converter generates active power= P positive
  note: Iq negative --> The converter generates reactive power ("Capacitive mode") = Q positive
  note: Sign Convention: Current going out of the converter = positive current
  note: Current Regulator
      | (with feedforward)
  note: Vq_sys + Id*w*L + Iq*R + deriv(Iq)*L= Vq_conv
  note: Vd_sys + Id*R - Iq*w*L + deriv(Id)*L= Vd_conv
  note: (Note: Derivative terms replaced by PI controllers)
  note: Vsys
  note: o-------
  note: I
  IdIq_ref : Inport  PortDimensions=2
  VdVq : Inport  Port=2  PortDimensions=2
  Freq : Inport  Port=3  PortDimensions=1
  wt : Inport  Port=4  PortDimensions=1
  IdIq : Inport  Port=5  PortDimensions=2
  Vdc : Inport  Port=6  PortDimensions=1
  " (Hz)" : Constant  Value=Vnom_dc  SampleTime=Ts
  Add1 : Sum  Inputs=+++-
  Add3 : Sum  Inputs=++++
  Avoid division by zero1 : Saturate  UpperLimit=Vnom_dc*1.25  LowerLimit=Vnom_dc*0.75
  Constant1 : Constant  Value=Lff  SampleTime=Ts_Control
  Constant2 : Constant  Value=Lff  SampleTime=Ts_Control
  Constant3 : Constant  Value=0  SampleTime=Ts
  Demux : Demux  Commented=on  Outputs=2
  Demux1 : Demux  Outputs=2
  Demux2 : Demux  Outputs=2
  Demux3 : Demux  Outputs=2
  Divide : Product  Inputs=*/
  Divide1 : Product  Inputs=**
  Gain : Gain  Gain=Rff
  Gain1 : Gain  Gain=Rff
  Math Function : Math  Commented=on  Operator=hypot  SignedPower=on
  Mean : spsMeanLib/Mean  Freq=Fnom/3  Vinit=Vnom_dc  Ts=Ts
  Mux : Mux  Inputs=2
  Mux1 : Mux  Inputs=2
  Mux2 : Mux  Inputs=[2 1]
  PI regulator with anti-windup D : Subsystem  DialogController=POWERSYS.PowerSysDialog  mask(Discrete PI Controller){Kp=Kp_Ireg, Ki=Ki_Ireg, Par_Limits=Limits_Ireg, Init=0, Ts=Ts}
      mask prompts: Kp "Proportional gain (Kp):"; Ki "Integral gain (Ki):"; Par_Limits "Output limits: [ Upper   Lower ]"; Init "Output initial value:"; Ts "Sample time:"
      mask help: This block implements a discrete PI controller.
      mask init:
      | UpperLimit=Par_Limits(1);
      | LowerLimit=Par_Limits(2);
      | power_initmask();
      mask Help: This block is part of a subset of blocks in the Extras library that does not have documentation associated with it, other than the block mask description.
      mask Display: disp('PI');
  PI regulator with anti-windup Q : Subsystem  DialogController=POWERSYS.PowerSysDialog  mask(Discrete PI Controller){Kp=Kp_Ireg, Ki=Ki_Ireg, Par_Limits=Limits_Ireg, Init=0, Ts=Ts}
      mask prompts: Kp "Proportional gain (Kp):"; Ki "Integral gain (Ki):"; Par_Limits "Output limits: [ Upper   Lower ]"; Init "Output initial value:"; Ts "Sample time:"
      mask help: This block implements a discrete PI controller.
      mask init:
      | UpperLimit=Par_Limits(1);
      | LowerLimit=Par_Limits(2);
      | power_initmask();
      mask Help: This block is part of a subset of blocks in the Extras library that does not have documentation associated with it, other than the block mask description.
      mask Display: disp('PI');
  Product1 : Product  Inputs=3  RndMeth=Zero
  Product2 : Product  Inputs=3  RndMeth=Zero
  Rtot_pu3 : Gain  Gain=1/Fnom  SaturateOnIntegerOverflow=on  OutDataTypeStr=Inherit: Same as input  ParamDataTypeStr=Inherit: Same as input
  Saturation : Saturate  UpperLimit=Limits_Ireg(1)  LowerLimit=Limits_Ireg(2)
  Sum : Sum  Inputs=|-+
  Sum1 : Sum  Inputs=|-+
  dq0 to abc : spsdq0toabcLib/dq0 to abc  Alignment=90 degrees behind phase A axis
  to-pu : Gain  Gain=1/(Vnom_dc/2*sqrt(3)/sqrt(2)/Vnom_sec)
  Uref_ABC : Outport
  m : Outport  Port=2
  PIdq : Outport  Port=3
  wires:
  wt/1 -> dq0 to abc/2
  to-pu/1 -> Saturation/1
  Mux/1 -> Divide1/1
  dq0 to abc/1 -> Uref_ABC/1
  Divide/1 -> Divide1/2
  Mean/1 -> Avoid division by zero1/1
  Divide1/1 -> to-pu/1
  " (Hz)"/1 -> Divide/1
  Vdc/1 -> Mean/1
  Avoid division by zero1/1 -> Divide/2
  Mux1/1 -> PIdq/1
  Constant3/1 -> Mux2/2
  Mux2/1 -> dq0 to abc/1
  Demux/2 -> Math Function/2
  Demux/1 -> Math Function/1
  Saturation/1 -> Mux2/1, m/1, Demux/1
  PI regulator with anti-windup D/1(Out) -> [PId], Add1/2
  PI regulator with anti-windup Q/1(Out) -> [PIq], Add3/2
  [Vd] -> Add1/1
  Product1/1 -> Add1/4
  Gain/1 -> Add1/3
  Gain1/1 -> Add3/3
  Product2/1 -> Add3/4
  [Vq] -> Add3/1
  Demux2/1 -> [Id]
  IdIq/1 -> Demux2/1
  [Id_ref] -> Product2/1
  [Iq_ref] -> Gain1/1
  [Iq_ref] -> Product1/1
  [Id_ref] -> Gain/1
  [Id] -> Sum/1
  [Iq] -> Sum1/1
  Demux2/2 -> [Iq]
  [PIq] -> Mux1/2
  [PId] -> Mux1/1
  [w] -> Product1/3
  Constant2/1 -> Product1/2
  [w] -> Product2/3
  Constant1/1 -> Product2/2
  [Iq_ref] -> Sum1/2
  Sum1/1 -> PI regulator with anti-windup Q/1(Error)
  [Id_ref] -> Sum/2
  Sum/1 -> PI regulator with anti-windup D/1(Error)
  VdVq/1 -> Demux3/1
  Demux3/2 -> [Vq]
  Demux3/1 -> [Vd]
  IdIq_ref/1 -> Demux1/1
  Demux1/2 -> [Iq_ref]
  Demux1/1 -> [Id_ref]
  Rtot_pu3/1 -> [w]
  Freq/1 -> Rtot_pu3/1
  Add1/1 -> Mux/1
  Add3/1 -> Mux/2

== system 20240109_HVDCMMCInterconnection/Control2/DC Voltage Regulator (VDCreg) ==
  note: VDC Regulator
  Vdc_ref : Inport  PortDimensions=1
  On : Inport  Port=2  PortDimensions=1
  Vdc_meas : Inport  Port=3  PortDimensions=1
  Discrete-Time Integrator : DiscreteIntegrator  SampleTime=Ts  LimitOutput=on  UpperSaturationLimit=Limits_VDCreg(1)  LowerSaturationLimit=Limits_VDCreg(2)  ICPrevOutput=DiscIntNeverNeededParam  ICPrevScaledInput=DiscIntNeverNeededParam
  Product : Product  RndMeth=Zero
  Product1 : Product  RndMeth=Zero
  Rtot_pu2 : Gain  Gain=1/Vnom_dc  SaturateOnIntegerOverflow=on  OutDataTypeStr=Inherit: Same as input  ParamDataTypeStr=Inherit: Same as input
  Saturation2 : Saturate  UpperLimit=Limits_VDCreg(1)  LowerLimit=Limits_VDCreg(2)  SampleTime=Ts
  Sum : Sum  Inputs=|+-
  Sum6 : Sum  InputSameDT=on  SaturateOnIntegerOverflow=on  SampleTime=Ts  OutDataTypeStr=Inherit: Same as first input
  Switch1 : Switch  Criteria=u2 ~= 0  Threshold=0.5  OutDataTypeStr=double  SaturateOnIntegerOverflow=off  InputSameDT=off
  VdcNom_SM : Constant  Value=Kp_VDCreg
  VdcNom_SM1 : Constant  Value=Ki_VDCreg
  Zero-Order Hold : ZeroOrderHold  SampleTime=Ts
  Id_ref : Outport
  wires:
  Rtot_pu2/1 -> Product/2, Product1/2
  Saturation2/1 -> Id_ref/1
  VdcNom_SM/1 -> Product1/1
  Product/1 -> Discrete-Time Integrator/1
  Product1/1 -> Zero-Order Hold/1
  VdcNom_SM1/1 -> Product/1
  Sum6/1 -> Saturation2/1
  Discrete-Time Integrator/1 -> Sum6/2
  Zero-Order Hold/1 -> Sum6/1
  Vdc_ref/1 -> Sum/2, Switch1/3
  Switch1/1 -> Sum/1
  On/1 -> Switch1/2
  Sum/1 -> Rtot_pu2/1
  Vdc_meas/1 -> Switch1/1

== system 20240109_HVDCMMCInterconnection/Control2/PLL, Measurements and Transformation ==
  note: P (pu) = Vd*Id + Vq*Iq
  note: Q (pu) = Vq*Id - Vd*Iq
  note: P positive = Converter generates active power (Inverter Mode)
  note: Q positive = Converter generates reactive power (Capacitive Mode)
  Vabc : Inport  PortDimensions=3
  Iabc : Inport  Port=2  PortDimensions=3
  Add : Sum  Inputs=1
  Demux : Demux  Outputs=2
  Discrete Mean value : powerlib_extras/Discrete Measurements/Discrete  Mean value  Freq=Fnom  Vinit=0  Ts=Ts
  Discrete Mean value1 : powerlib_extras/Discrete Measurements/Discrete  Mean value  Freq=Fnom  Vinit=0  Ts=Ts
  I->pu2 : Gain  Gain=sqrt(3)*Vnom_sec/sqrt(2)/Pnom  SaturateOnIntegerOverflow=on  OutDataTypeStr=Inherit: Same as input  ParamDataTypeStr=Inherit: Same as input
  PLL (3ph) : spsPLL3phLib/PLL (3ph)  Fmin=0.9*Fnom  Par_Init=[0, Fnom]  ParK=[180, 3200, 1]  TcD=1e-4  MaxRateChangeFreq=12  FilterCutOffFreq=25  Ts=Ts  AGC=on
  Product : Product  RndMeth=Zero
  Product1 : Product  RndMeth=Zero
  Second-Order Filter : spsSecondOrderFilterLib/Second-Order Filter  FilterType=Lowpass  Fo=Fn_filter  Zeta=Zeta_filter  Ts=Ts  Initialize=off  Vac_Init="[0,  0,  60]"  Vdc_Init=0  PlotResponse=off  FreqRange=[0, 500, 1]
  Second-Order Filter1 : spsSecondOrderFilterLib/Second-Order Filter  FilterType=Lowpass  Fo=Fn_filter  Zeta=Zeta_filter  Ts=Ts  Initialize=off  Vac_Init="[0,  0,  60]"  Vdc_Init=0  PlotResponse=off  FreqRange=[0, 500, 1]
  Selector3 : Selector  InputPortWidth=2  IndexOptions=Index vector (dialog)  Indices=[2 1]  OutputSizes=1
  Selector4 : Selector  InputPortWidth=3  IndexOptions=Index vector (dialog)  Indices=[1 2]  OutputSizes=1
  Selector5 : Selector  InputPortWidth=3  IndexOptions=Index vector (dialog)  Indices=[1 2]  OutputSizes=1
  Subtract : Sum  Inputs=+-
  V->pu1 : Gain  Gain=1/(Vnom_sec/sqrt(3)*sqrt(2))  SaturateOnIntegerOverflow=on  OutDataTypeStr=Inherit: Same as input  ParamDataTypeStr=Inherit: Same as input
  abc to dq0 : spsabctodq0Lib/abc to dq0  Alignment=90 degrees behind phase A axis
  abc to dq1 : spsabctodq0Lib/abc to dq0  Alignment=90 degrees behind phase A axis
  Freq : Outport
  wt : Outport  Port=2
  IdIq : Outport  Port=3
  P : Outport  Port=4
  Q : Outport  Port=5
  VdVq : Outport  Port=6
  wires:
  Selector3/1 -> Product1/1
  Discrete Mean value1/1 -> Q/1
  Discrete Mean value/1 -> P/1
  Second-Order Filter/1 -> VdVq/1, Product/1, Selector3/1
  Second-Order Filter1/1 -> IdIq/1, Product1/2, Product/2
  Product/1 -> Add/1
  Product1/1 -> Demux/1
  Demux/1 -> Subtract/1
  Demux/2 -> Subtract/2
  Add/1 -> Discrete Mean value/1
  Subtract/1 -> Discrete Mean value1/1
  abc to dq0/1 -> Selector4/1
  PLL (3ph)/1 -> Freq/1
  V->pu1/1 -> abc to dq0/1, PLL (3ph)/1
  Vabc/1 -> V->pu1/1
  PLL (3ph)/2 -> wt/1, abc to dq1/2, abc to dq0/2
  Iabc/1 -> I->pu2/1
  abc to dq1/1 -> Selector5/1
  I->pu2/1 -> abc to dq1/1
  Selector4/1 -> Second-Order Filter/1
  Selector5/1 -> Second-Order Filter1/1

== system 20240109_HVDCMMCInterconnection/Control2/Reactive Power Regulator ==
  note: Reactive Power Regulator
  note: If PLL sync on Vprim --> Vq=0 --> Id = P/Vd et Iq = -1.0 * Q/Vd
  note: Q (pu) = Vq*Id - Vd*Iq (valid only for balanced & harmonics-free values)
  note: P (pu) = Vd*Id + Vq*Iq (Zero-sequence is not taken into account)
  On : Inport  PortDimensions=1
  Qref : Inport  Port=2  PortDimensions=1
  Qmes : Inport  Port=3  PortDimensions=1
  VdVq_mes : Inport  Port=4  PortDimensions=2
  Add2 : Sum
  Discrete Mean value1 : powerlib_extras/Discrete Measurements/Discrete  Mean value  Freq=Fnom  Vinit=0  Ts=Ts
  Discrete-Time Integrator : DiscreteIntegrator  SampleTime=Ts  LimitOutput=on  UpperSaturationLimit=Limits_Qreg(1)  LowerSaturationLimit=Limits_Qreg(2)  ICPrevOutput=DiscIntNeverNeededParam  ICPrevScaledInput=DiscIntNeverNeededParam
  Divide : Product  Inputs=*/
  Product : Product  RndMeth=Zero
  Product1 : Product  RndMeth=Zero
  Rtot_pu1 : Gain  Gain=-1  SaturateOnIntegerOverflow=on  OutDataTypeStr=Inherit: Same as input  ParamDataTypeStr=Inherit: Same as input
  Rtot_pu2 : Gain  Gain=-1  SaturateOnIntegerOverflow=on  OutDataTypeStr=Inherit: Same as input  ParamDataTypeStr=Inherit: Same as input
  Saturation : Saturate  UpperLimit=Limits_Qreg(1)  LowerLimit=Limits_Qreg(2)
  Saturation1 : Saturate  UpperLimit=2  LowerLimit=1e-6
  Saturation2 : Saturate  UpperLimit=Limits_Qreg(1)  LowerLimit=Limits_Qreg(2)
  Selector : Selector  InputPortWidth=2  IndexOptions=Index vector (dialog)  Indices=[1]  OutputSizes=1
  Sum : Sum  Inputs=|-+
  Sum6 : Sum  InputSameDT=on  SaturateOnIntegerOverflow=on  SampleTime=Ts  OutDataTypeStr=Inherit: Same as first input
  Switch1 : Switch  Criteria=u2 ~= 0  Threshold=0.5  OutDataTypeStr=double  SaturateOnIntegerOverflow=off  InputSameDT=off
  VdcNom_SM : Constant  Value=Kp_Qreg
  VdcNom_SM1 : Constant  Value=Ki_Qreg
  Zero-Order Hold : ZeroOrderHold  SampleTime=Ts
  Iq_ref : Outport
  wires:
  Saturation2/1 -> Rtot_pu1/1
  Saturation/1 -> Iq_ref/1
  Rtot_pu2/1 -> Add2/2
  Rtot_pu1/1 -> Add2/1
  Sum6/1 -> Saturation2/1
  Switch1/1 -> Product1/2, Product/2
  Sum/1 -> Switch1/1
  On/1 -> Switch1/2
  Add2/1 -> Saturation/1
  Product/1 -> Discrete-Time Integrator/1
  Product1/1 -> Zero-Order Hold/1
  VdcNom_SM/1 -> Product1/1
  VdcNom_SM1/1 -> Product/1
  Discrete-Time Integrator/1 -> Sum6/2
  Zero-Order Hold/1 -> Sum6/1
  Discrete Mean value1/1 -> Saturation1/1
  Saturation1/1 -> Divide/2
  Divide/1 -> Rtot_pu2/1
  Selector/1 -> Discrete Mean value1/1
  VdVq_mes/1 -> Selector/1
  Qmes/1 -> Sum/1
  Qref/1 -> Divide/1, Switch1/3, Sum/2

== system 20240109_HVDCMMCInterconnection/Control3/Active Power Regulator (Preg) ==
  note: Active Power Regulator
  Pmeas : Inport  PortDimensions=1
  Pref : Inport  Port=2  PortDimensions=1  SampleTime=Ts
  On : Inport  Port=3  PortDimensions=1  SampleTime=Ts
  Discrete-Time Integrator : DiscreteIntegrator  InitialCondition=1  SampleTime=Ts  LimitOutput=on  UpperSaturationLimit=Limits_Preg(1)  LowerSaturationLimit=Limits_Preg(2)  ICPrevOutput=DiscIntNeverNeededParam  ICPrevScaledInput=DiscIntNeverNeededParam
  Product : Product  RndMeth=Zero
  Product1 : Product  RndMeth=Zero
  Product2 : Product
  Saturation2 : Saturate  UpperLimit=Limits_Preg(1)  LowerLimit=Limits_Preg(2)  SampleTime=Ts
  Sum : Sum  Inputs=|+-
  Sum6 : Sum  InputSameDT=on  SaturateOnIntegerOverflow=on  SampleTime=Ts  OutDataTypeStr=Inherit: Same as first input
  Switch1 : Switch  Criteria=u2 ~= 0  Threshold=0.5  OutDataTypeStr=double  SaturateOnIntegerOverflow=off  InputSameDT=off
  VdcNom_SM : Constant  Value=Kp_Preg  SampleTime=Ts
  VdcNom_SM1 : Constant  Value=Ki_Preg  SampleTime=Ts
  VdcNom_SM2 : Constant  Value=Vnom_dc  SampleTime=Ts
  Zero-Order Hold : ZeroOrderHold  SampleTime=Ts
  Vdc_ref : Outport  SampleTime=Ts
  wires:
  Product2/1 -> Vdc_ref/1
  VdcNom_SM2/1 -> Product2/2
  Pmeas/1 -> Switch1/1
  On/1 -> Switch1/2
  Switch1/1 -> Sum/1
  Pref/1 -> Switch1/3, Sum/2
  Zero-Order Hold/1 -> Sum6/1
  Discrete-Time Integrator/1 -> Sum6/2
  Sum6/1 -> Saturation2/1
  VdcNom_SM1/1 -> Product/1
  Product1/1 -> Zero-Order Hold/1
  Product/1 -> Discrete-Time Integrator/1
  VdcNom_SM/1 -> Product1/1
  Saturation2/1 -> Product2/1
  Sum/1 -> Product1/2, Product/2
